simulink model "rectify1"  (R2018b)
settings: Solver=VariableStepAuto  StartTime=0.0  StopTime=10.0  RelTol=1e-3
settings Model: Creator=Control System Lab  LastModifiedBy=Control System Lab

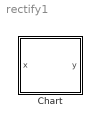
== system rectify1 ==
  Chart : Stateflow chart  TreatAsAtomicUnit=on

== stateflow chart rectify1/Chart ==
  state On
    y=x;
  state Off
    y=0;
  (default) -> On
  Off -> On : [x<t0]
  On -> Off : [x>=t0]
  data: x input; y output; t0 constant double =0
